simulink model "assignmnet8model"  (R2015a)
settings: Solver=ode45  StartTime=0.0  StopTime=time(end)  RelTol=1e-3
model workspace: external: MATLAB File C:\Users\kate\Documents\MATLAB\Assign8.m (data not in the file)
values from neighbouring files (symbols this model uses):
  area = 20    [Assign8.m]
  max_output = 10    [Assign8.m]
  pcoef5 = [7.79e-05,-0.0032,0.0385,-0.05,-.014,0.09]    [Assign8.m]
settings Model: Creator=kate  LastModifiedBy=kate
settings DataIOCC: ExternalInput=[time, windspeed, solarpower]  LoadExternalInput=on

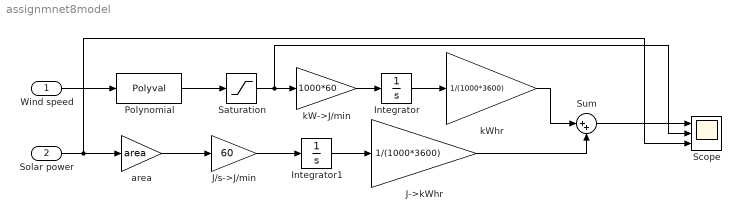
== system assignmnet8model ==
  Wind speed : Inport
  Solar power : Inport  Port=2
  Integrator : Integrator
  Integrator1 : Integrator
  J->kWhr : Gain  Gain=1/(1000*3600)
  J/s->J/min : Gain  Gain=60
  Polynomial : Polyval  Coefs=pcoef5
  Saturation : Saturate  UpperLimit=max_output  LowerLimit=0  OutMax=[10]
  Scope : Scope  NumInputPorts=3
      settings: YMin=-5~-5~-5  YMax=5~5~5
  Sum : Sum  Inputs=|++
  area : Gain  Gain=area
  kW->J/min : Gain  Gain=1000*60
  kWhr : Gain  Gain=1/(1000*3600)
  wires:
  Wind speed/1 -> Polynomial/1
  Polynomial/1 -> Saturation/1
  Saturation/1 -> Scope/2, kW->J/min/1
  kW->J/min/1 -> Integrator/1
  Integrator/1 -> kWhr/1
  kWhr/1 -> Sum/1
  area/1 -> J/s->J/min/1
  Integrator1/1 -> J->kWhr/1
  J/s->J/min/1 -> Integrator1/1
  J->kWhr/1 -> Sum/2
  Solar power/1 -> Scope/3, area/1
  Sum/1 -> Scope/1
